simulink model "Two_Zone_MVDC_PSolver_R2020b"  (R2020b)
settings: Solver=FixedStepDiscrete  StartTime=0.0  StopTime=30  FixedStep=TsELEC  RelTol=1e-3  EnableMultiTasking=on
InitFcn:
  | TsELEC = 25e-6;
  | Ts = 25e-6;
  | TsTHERMAL = 1e-3;
  | TsCont = TsELEC;
  | Rsnub = 1e4;
undefined symbols (not defined in the file or in its folder): DiscIntNeverNeededParam, ee_sli_rtmsupport, GABDA, GABDB, GBBDA, GBBDB, gcbh, GPMMA, GPPMB, GPPMC, SADA, SADB, SADC, SADD, SBDA, SBDB, SBDC, SCDA, SCDB, SCDC, SCDD, SDDA, SDDB, SDDC, SDDD, SDDE
libraries: fl_lib x138, nesl_utility x69, ee_lib x52, simulink x3, pid_lib x3, eeTransforms x3, sps_avr x2, powerlib_meascontrol x2, slrealtimetgmanagement x1
(part 1 of 4)
settings Model: SimulationMode=accelerator  Creator=gdudgeon  LastModifiedBy=gdudgeon
settings SolverCC: ConcurrentTasks=on  PositivePriorityOrder=on  AutoInsertRateTranBlk=on
settings DataIOCC: SaveFormat=StructureWithTime  SaveOutput=off  DSMLogging=off  SaveTime=off  ReturnWorkspaceOutputs=off
settings OptimizationCC: BlockReduction=off  OptimizeBlockIOStorage=off  BufferReuse=off  GlobalBufferReuse=off  ExpressionFolding=off  LocalBlockOutputs=off  OptimizeDataStoreBuffers=off  BusAssignmentInplaceUpdate=off
settings HardwareCC: ProdBitPerLong=64  ProdLongLongMode=on  ProdHWDeviceType=Intel->x86-64 (Linux 64)
settings ModelReferenceCC: ModelReferenceNumInstancesAllowed=Single  ModelReferenceMinAlgLoopOccurrences=on
settings SFSimCC: CustomCodeUndefinedFunction=UseInterfaceOnly
settings RTWCC: Description=Simulink Real-Time  SystemTargetFile=slrealtime.tlc  TLCOptions=-axPCMaxOverloads=300  TemplateMakefile=slrealtime_default_tmf  Toolchain=Simulink Real-Time Toolchain  BuildConfiguration=Faster Runs  CodeExecutionProfiling=on  TargetLang=C++

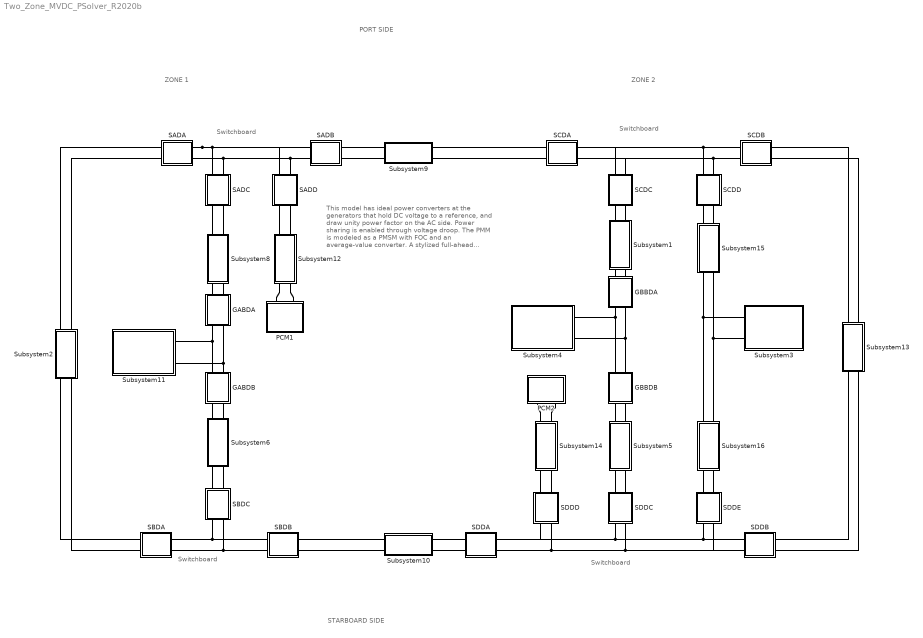
== system Two_Zone_MVDC_PSolver_R2020b ==
  note: This model has ideal power converters at the generators that hold DC voltage to a reference, and draw unity power factor on the AC side. Power sharing is enabled through voltage droop.
      |
      | The PMM is modeled as a PMSM with FOC and an average-value converter.
      |
      | A stylized full-ahead crash-stop maneuver with quadrant II regeneration is simulated.
      |
      | The model uses snubbers on the inductive lines to enable the use of partitioning solver.
  note: PORT SIDE
  note: Switchboard
  note: ZONE 1
  note: ZONE 2
  note: Switchboard
  note: Switchboard
  note: Switchboard
  note: STARBOARD SIDE
  GABDA : Subsystem  mask{status=GABDA}
      mask prompts: status "Initial Status"
      mask init:
      | if ~status
      |     
      |     set(gcbh,'BackgroundColor','green')
      |     
      | elseif status
      |     
      |     set(gcbh,'BackgroundColor','red')
      |     
      | end
  GABDB : Subsystem  mask{status=GABDB}
      mask prompts: status "Initial Status"
      mask init:
      | if ~status
      |     
      |     set(gcbh,'BackgroundColor','green')
      |     
      | elseif status
      |     
      |     set(gcbh,'BackgroundColor','red')
      |     
      | end
  GBBDA : Subsystem  mask{status=GBBDA}
      mask prompts: status "Initial Status"
      mask init:
      | if ~status
      |     
      |     set(gcbh,'BackgroundColor','green')
      |     
      | elseif status
      |     
      |     set(gcbh,'BackgroundColor','red')
      |     
      | end
  GBBDB : Subsystem  mask{status=GBBDB}
      mask prompts: status "Initial Status"
      mask init:
      | if ~status
      |     
      |     set(gcbh,'BackgroundColor','green')
      |     
      | elseif status
      |     
      |     set(gcbh,'BackgroundColor','red')
      |     
      | end
  PCM1 : Subsystem
      mask Display: disp('PCM1')
  PCM2 : Subsystem
      mask Display: disp('PCM2')
  SADA : Subsystem  mask{status=SADA}
      mask prompts: status "Initial Status"
      mask init:
      | if ~status
      |     
      |     set(gcbh,'BackgroundColor','green')
      |     
      | elseif status
      |     
      |     set(gcbh,'BackgroundColor','red')
      |     
      | end
  SADB : Subsystem  mask{status=SADB}
      mask prompts: status "Initial Status"
      mask init:
      | if ~status
      |     
      |     set(gcbh,'BackgroundColor','green')
      |     
      | elseif status
      |     
      |     set(gcbh,'BackgroundColor','red')
      |     
      | end
  SADC : Subsystem  mask{status=SADC}
      mask prompts: status "Initial Status"
      mask init:
      | if ~status
      |     
      |     set(gcbh,'BackgroundColor','green')
      |     
      | elseif status
      |     
      |     set(gcbh,'BackgroundColor','red')
      |     
      | end
  SADD : Subsystem  mask{status=SADD}
      mask prompts: status "Initial Status"
      mask init:
      | if ~status
      |     
      |     set(gcbh,'BackgroundColor','green')
      |     
      | elseif status
      |     
      |     set(gcbh,'BackgroundColor','red')
      |     
      | end
  SBDA : Subsystem  mask{status=SBDA}
      mask prompts: status "Initial Status"
      mask init:
      | if ~status
      |     
      |     set(gcbh,'BackgroundColor','green')
      |     
      | elseif status
      |     
      |     set(gcbh,'BackgroundColor','red')
      |     
      | end
  SBDB : Subsystem  mask{status=SBDB}
      mask prompts: status "Initial Status"
      mask init:
      | if ~status
      |     
      |     set(gcbh,'BackgroundColor','green')
      |     
      | elseif status
      |     
      |     set(gcbh,'BackgroundColor','red')
      |     
      | end
  SBDC : Subsystem  mask{status=SBDC}
      mask prompts: status "Initial Status"
      mask init:
      | if ~status
      |     
      |     set(gcbh,'BackgroundColor','green')
      |     
      | elseif status
      |     
      |     set(gcbh,'BackgroundColor','red')
      |     
      | end
  SCDA : Subsystem  mask{status=SCDA}
      mask prompts: status "Initial Status"
      mask init:
      | if ~status
      |     
      |     set(gcbh,'BackgroundColor','green')
      |     
      | elseif status
      |     
      |     set(gcbh,'BackgroundColor','red')
      |     
      | end
  SCDB : Subsystem  mask{status=SCDB}
      mask prompts: status "Initial Status"
      mask init:
      | if ~status
      |     
      |     set(gcbh,'BackgroundColor','green')
      |     
      | elseif status
      |     
      |     set(gcbh,'BackgroundColor','red')
      |     
      | end
  SCDC : Subsystem  mask{status=SCDC}
      mask prompts: status "Initial Status"
      mask init:
      | if ~status
      |     
      |     set(gcbh,'BackgroundColor','green')
      |     
      | elseif status
      |     
      |     set(gcbh,'BackgroundColor','red')
      |     
      | end
  SCDD : Subsystem  mask{status=SCDD}
      mask prompts: status "Initial Status"
      mask init:
      | if ~status
      |     
      |     set(gcbh,'BackgroundColor','green')
      |     
      | elseif status
      |     
      |     set(gcbh,'BackgroundColor','red')
      |     
      | end
  SDDA : Subsystem  mask{status=SDDA}
      mask prompts: status "Initial Status"
      mask init:
      | if ~status
      |     
      |     set(gcbh,'BackgroundColor','green')
      |     
      | elseif status
      |     
      |     set(gcbh,'BackgroundColor','red')
      |     
      | end
  SDDB : Subsystem  mask{status=SDDB}
      mask prompts: status "Initial Status"
      mask init:
      | if ~status
      |     
      |     set(gcbh,'BackgroundColor','green')
      |     
      | elseif status
      |     
      |     set(gcbh,'BackgroundColor','red')
      |     
      | end
  SDDC : Subsystem  mask{status=SDDC}
      mask prompts: status "Initial Status"
      mask init:
      | if ~status
      |     
      |     set(gcbh,'BackgroundColor','green')
      |     
      | elseif status
      |     
      |     set(gcbh,'BackgroundColor','red')
      |     
      | end
  SDDD : Subsystem  mask{status=SDDD}
      mask prompts: status "Initial Status"
      mask init:
      | if ~status
      |     
      |     set(gcbh,'BackgroundColor','green')
      |     
      | elseif status
      |     
      |     set(gcbh,'BackgroundColor','red')
      |     
      | end
  SDDE : Subsystem  mask{status=SDDE}
      mask prompts: status "Initial Status"
      mask init:
      | if ~status
      |     
      |     set(gcbh,'BackgroundColor','green')
      |     
      | elseif status
      |     
      |     set(gcbh,'BackgroundColor','red')
      |     
      | end
  Subsystem1 : Subsystem
      mask Display: disp('CS11*')
  Subsystem10 : Subsystem
      mask Display: disp('CS6')
  Subsystem11 : Subsystem
      mask Display: disp('PGM1')
  Subsystem12 : Subsystem
      mask Display: disp('CS21')
  Subsystem13 : Subsystem
      mask Display: disp('CS4')
  Subsystem14 : Subsystem
      mask Display: disp('CS22')
  Subsystem15 : Subsystem
      mask Display: disp('CS14*')
  Subsystem16 : Subsystem
      mask Display: disp('CS14')
  Subsystem2 : Subsystem
      mask Display: disp('CS8')
  Subsystem3 : Subsystem
      mask Display: disp('PMM')
  Subsystem4 : Subsystem
      mask Display: disp('PGM2')
  Subsystem5 : Subsystem
      mask Display: disp('CS11')
  Subsystem6 : Subsystem
      mask Display: disp('CS9*')
  Subsystem8 : Subsystem
      mask Display: disp('CS9')
  Subsystem9 : Subsystem
      mask Display: disp('CS2')
  connections:
  SADA/RConn2 -- SADC/LConn2 -- SADD/LConn2 -- SADB/LConn2
  SBDC/RConn2 -- SBDB/LConn2 -- SBDA/RConn2
  Subsystem11/RConn2 -- GABDB/LConn2 -- GABDA/RConn2
  Subsystem11/RConn1 -- GABDB/LConn1 -- GABDA/RConn1
  SADA/RConn1 -- SADD/LConn1 -- SADB/LConn1 -- SADC/LConn1
  SBDC/RConn1 -- SBDB/LConn1 -- SBDA/RConn1
  SCDA/LConn2 -- Subsystem9/LConn2
  SADB/RConn1 -- Subsystem9/RConn1
  Subsystem12/LConn1 -- SADD/RConn1
  SBDA/LConn2 -- Subsystem2/RConn2
  SBDC/LConn1 -- Subsystem6/RConn1
  Subsystem12/RConn1 -- PCM1/LConn1
  SBDB/RConn1 -- Subsystem10/RConn1
  SBDC/LConn2 -- Subsystem6/RConn2
  Subsystem2/LConn1 -- SADA/LConn1
  Subsystem12/RConn2 -- PCM1/LConn2
  Subsystem12/LConn2 -- SADD/RConn2
  SADC/RConn1 -- Subsystem8/LConn1
  SBDB/RConn2 -- Subsystem10/RConn2
  SADB/RConn2 -- Subsystem9/RConn2
  Subsystem2/LConn2 -- SADA/LConn2
  SBDA/LConn1 -- Subsystem2/RConn1
  SADC/RConn2 -- Subsystem8/LConn2
  GBBDA/RConn1 -- GBBDB/LConn1 -- Subsystem4/RConn1
  SDDC/RConn2 -- SDDB/LConn2 -- SDDE/RConn2 -- SDDA/RConn2 -- SDDD/RConn2
  SCDC/LConn2 -- SCDA/RConn2 -- SCDD/LConn2 -- SCDB/LConn2
  SDDC/RConn1 -- SDDA/RConn1 -- SDDD/RConn1 -- SDDB/LConn1 -- SDDE/RConn1
  SCDC/LConn1 -- SCDA/RConn1 -- SCDD/LConn1 -- SCDB/LConn1
  GBBDA/RConn2 -- GBBDB/LConn2 -- Subsystem4/RConn2
  SCDC/RConn2 -- Subsystem1/LConn2
  SCDB/RConn1 -- Subsystem13/LConn1
  SDDB/RConn1 -- Subsystem13/RConn1
  SDDC/LConn2 -- Subsystem5/RConn2
  SDDB/RConn2 -- Subsystem13/RConn2
  SCDB/RConn2 -- Subsystem13/LConn2
  SDDC/LConn1 -- Subsystem5/RConn1
  SCDC/RConn1 -- Subsystem1/LConn1
  Subsystem9/LConn1 -- SCDA/LConn1
  Subsystem10/LConn1 -- SDDA/LConn1
  Subsystem10/LConn2 -- SDDA/LConn2
  GBBDA/LConn1 -- Subsystem1/RConn1
  GBBDA/LConn2 -- Subsystem1/RConn2
  GBBDB/RConn1 -- Subsystem5/LConn1
  GBBDB/RConn2 -- Subsystem5/LConn2
  GABDA/LConn1 -- Subsystem8/RConn1
  GABDA/LConn2 -- Subsystem8/RConn2
  GABDB/RConn1 -- Subsystem6/LConn1
  GABDB/RConn2 -- Subsystem6/LConn2
  Subsystem14/LConn1 -- PCM2/LConn1
  Subsystem14/LConn2 -- PCM2/LConn2
  Subsystem14/RConn1 -- SDDD/LConn1
  Subsystem14/RConn2 -- SDDD/LConn2
  Subsystem15/LConn2 -- SCDD/RConn2
  Subsystem15/LConn1 -- SCDD/RConn1
  Subsystem16/RConn1 -- SDDE/LConn1
  Subsystem16/RConn2 -- SDDE/LConn2
  Subsystem16/LConn1 -- Subsystem3/LConn1 -- Subsystem15/RConn1
  Subsystem15/RConn2 -- Subsystem16/LConn2 -- Subsystem3/LConn2

== system Two_Zone_MVDC_PSolver_R2020b/GABDA ==
  GABDA : ee_lib/Switches & Breakers/DPST Switch  R_closed=1e-4 Ohm  G_open=1e-6 S  Threshold=0.5 V  Width=0 V  model_dynamics=0  t_on=1e-3 s  t_off=1e-3 s  initial_vT=0 V
      settings: SourceProductBaseCode=PS  InternalSimscapePortConfiguration="{\"Bottom\":[],\"Left\":[{\"id\":\"vT\",\"label\":\"vT\",\"type\":\"input\"},{\"id\":\"p1\",\"label\":\"\",\"type\":\"foundation.electrical.electrical\"},{\"id\":\"p2\",\"label\":\"\",\"type\":\"foundation.electrical.electrical\"}],\"Right\":[{\"id\":\"n1\",\"label\":\"\",\"type\":\"foundation.electrical.electrical\"},{\"id\":\"n2\",\"label\":\"\",\"type\":\"foundation.electrical.electrical\"}],\"Top\":[]}"
  Simulink-PS Converter : nesl_utility/Simulink-PS Converter  PhysicalDomain=network_engine_domain  SubClassName=ps_input  LeftPortType=input  RightPortType=output  PseudoPeriodic=off  Frequencies=[]  NoiseDistribution=none  NoiseParameters=[]  Unit=1  AffineConversion=off  FilteringAndDerivatives=provide  SimscapeFilterOrder=1  InputFilterTimeConstant=0.001  UdotUserProvided=0
  "+ " : PMIOPort  Side=Right
  + : PMIOPort  Port=2  Side=Left
  "- " : PMIOPort  Port=3  Side=Right
  - : PMIOPort  Port=4  Side=Left
  wires:
  [GABDA] -> Simulink-PS Converter/1
  connections:
  GABDA/RConn1 -- "+ "/RConn1
  GABDA/LConn3 -- -/RConn1
  GABDA/RConn2 -- "- "/RConn1
  Simulink-PS Converter/RConn1 -- GABDA/LConn1
  GABDA/LConn2 -- +/RConn1

== system Two_Zone_MVDC_PSolver_R2020b/GABDB ==
  GABDB : ee_lib/Switches & Breakers/DPST Switch  R_closed=1e-4 Ohm  G_open=1e-6 S  Threshold=0.5 V  Width=0 V  model_dynamics=0  t_on=1e-3 s  t_off=1e-3 s  initial_vT=0 V
      settings: SourceProductBaseCode=PS  InternalSimscapePortConfiguration="{\"Bottom\":[],\"Left\":[{\"id\":\"vT\",\"label\":\"vT\",\"type\":\"input\"},{\"id\":\"p1\",\"label\":\"\",\"type\":\"foundation.electrical.electrical\"},{\"id\":\"p2\",\"label\":\"\",\"type\":\"foundation.electrical.electrical\"}],\"Right\":[{\"id\":\"n1\",\"label\":\"\",\"type\":\"foundation.electrical.electrical\"},{\"id\":\"n2\",\"label\":\"\",\"type\":\"foundation.electrical.electrical\"}],\"Top\":[]}"
  Simulink-PS Converter : nesl_utility/Simulink-PS Converter  PhysicalDomain=network_engine_domain  SubClassName=ps_input  LeftPortType=input  RightPortType=output  PseudoPeriodic=off  Frequencies=[]  NoiseDistribution=none  NoiseParameters=[]  Unit=1  AffineConversion=off  FilteringAndDerivatives=provide  SimscapeFilterOrder=1  InputFilterTimeConstant=0.001  UdotUserProvided=0
  "+ " : PMIOPort  Side=Right
  + : PMIOPort  Port=2  Side=Left
  "- " : PMIOPort  Port=3  Side=Right
  - : PMIOPort  Port=4  Side=Left
  wires:
  [GABDB] -> Simulink-PS Converter/1
  connections:
  GABDB/LConn2 -- +/RConn1
  Simulink-PS Converter/RConn1 -- GABDB/LConn1
  GABDB/RConn2 -- "- "/RConn1
  GABDB/LConn3 -- -/RConn1
  GABDB/RConn1 -- "+ "/RConn1

== system Two_Zone_MVDC_PSolver_R2020b/GBBDA ==
  GBBDA : ee_lib/Switches & Breakers/DPST Switch  R_closed=1e-4 Ohm  G_open=1e-6 S  Threshold=0.5 V  Width=0 V  model_dynamics=0  t_on=1e-3 s  t_off=1e-3 s  initial_vT=0 V
      settings: SourceProductBaseCode=PS  InternalSimscapePortConfiguration="{\"Bottom\":[],\"Left\":[{\"id\":\"vT\",\"label\":\"vT\",\"type\":\"input\"},{\"id\":\"p1\",\"label\":\"\",\"type\":\"foundation.electrical.electrical\"},{\"id\":\"p2\",\"label\":\"\",\"type\":\"foundation.electrical.electrical\"}],\"Right\":[{\"id\":\"n1\",\"label\":\"\",\"type\":\"foundation.electrical.electrical\"},{\"id\":\"n2\",\"label\":\"\",\"type\":\"foundation.electrical.electrical\"}],\"Top\":[]}"
  Simulink-PS Converter : nesl_utility/Simulink-PS Converter  PhysicalDomain=network_engine_domain  SubClassName=ps_input  LeftPortType=input  RightPortType=output  PseudoPeriodic=off  Frequencies=[]  NoiseDistribution=none  NoiseParameters=[]  Unit=1  AffineConversion=off  FilteringAndDerivatives=provide  SimscapeFilterOrder=1  InputFilterTimeConstant=0.001  UdotUserProvided=0
  "+ " : PMIOPort  Side=Right
  + : PMIOPort  Port=2  Side=Left
  "- " : PMIOPort  Port=3  Side=Right
  - : PMIOPort  Port=4  Side=Left
  wires:
  [GBBDA] -> Simulink-PS Converter/1
  connections:
  GBBDA/RConn1 -- "+ "/RConn1
  GBBDA/LConn3 -- -/RConn1
  GBBDA/RConn2 -- "- "/RConn1
  Simulink-PS Converter/RConn1 -- GBBDA/LConn1
  GBBDA/LConn2 -- +/RConn1

== system Two_Zone_MVDC_PSolver_R2020b/GBBDB ==
  GBBDB : ee_lib/Switches & Breakers/DPST Switch  R_closed=1e-4 Ohm  G_open=1e-6 S  Threshold=0.5 V  Width=0 V  model_dynamics=0  t_on=1e-3 s  t_off=1e-3 s  initial_vT=0 V
      settings: SourceProductBaseCode=PS  InternalSimscapePortConfiguration="{\"Bottom\":[],\"Left\":[{\"id\":\"vT\",\"label\":\"vT\",\"type\":\"input\"},{\"id\":\"p1\",\"label\":\"\",\"type\":\"foundation.electrical.electrical\"},{\"id\":\"p2\",\"label\":\"\",\"type\":\"foundation.electrical.electrical\"}],\"Right\":[{\"id\":\"n1\",\"label\":\"\",\"type\":\"foundation.electrical.electrical\"},{\"id\":\"n2\",\"label\":\"\",\"type\":\"foundation.electrical.electrical\"}],\"Top\":[]}"
  Simulink-PS Converter : nesl_utility/Simulink-PS Converter  PhysicalDomain=network_engine_domain  SubClassName=ps_input  LeftPortType=input  RightPortType=output  PseudoPeriodic=off  Frequencies=[]  NoiseDistribution=none  NoiseParameters=[]  Unit=1  AffineConversion=off  FilteringAndDerivatives=provide  SimscapeFilterOrder=1  InputFilterTimeConstant=0.001  UdotUserProvided=0
  "+ " : PMIOPort  Side=Right
  + : PMIOPort  Port=2  Side=Left
  "- " : PMIOPort  Port=3  Side=Right
  - : PMIOPort  Port=4  Side=Left
  wires:
  [GBBDB] -> Simulink-PS Converter/1
  connections:
  GBBDB/LConn2 -- +/RConn1
  Simulink-PS Converter/RConn1 -- GBBDB/LConn1
  GBBDB/RConn2 -- "- "/RConn1
  GBBDB/LConn3 -- -/RConn1
  GBBDB/RConn1 -- "+ "/RConn1

== system Two_Zone_MVDC_PSolver_R2020b/PCM1 ==
  Bus Creator : BusCreator  Inputs=3
  Current Sensor : fl_lib/Electrical/Electrical Sensors/Current Sensor
  PS-Simulink Converter : nesl_utility/PS-Simulink Converter  PhysicalDomain=network_engine_domain  SubClassName=ps_output  LeftPortType=input  RightPortType=output  PseudoPeriodic=off  Frequencies=[]  Unit=1  AffineConversion=off
  PS-Simulink Converter1 : nesl_utility/PS-Simulink Converter  PhysicalDomain=network_engine_domain  SubClassName=ps_output  LeftPortType=input  RightPortType=output  PseudoPeriodic=off  Frequencies=[]  Unit=1  AffineConversion=off
  Product : Product
  Resistor : fl_lib/Electrical/Electrical Elements/Resistor  R=100 Ohm  i_specify=off  i_priority=None  i=0 A  i_nominal_specify=off  i_nominal_unit=A  i_nominal_value=1  v_specify=off  v_priority=None  v=0 V  v_nominal_specify=off  v_nominal_unit=V  v_nominal_value=1
  Terminator : Terminator
  Voltage Sensor : fl_lib/Electrical/Electrical Sensors/Voltage Sensor
  + : PMIOPort  Side=Left
  - : PMIOPort  Port=2  Side=Left
  wires:
  Bus Creator/1 -> Terminator/1  "PCM1"
  Product/1 -> Bus Creator/3  "P"
  PS-Simulink Converter1/1 -> Bus Creator/2, Product/2  "V"
  PS-Simulink Converter/1 -> Bus Creator/1, Product/1  "I"
  connections:
  Current Sensor/LConn1 -- +/RConn1
  Voltage Sensor/RConn1 -- PS-Simulink Converter1/LConn1
  PS-Simulink Converter/LConn1 -- Current Sensor/RConn1
  Resistor/RConn1 -- -/RConn1 -- Voltage Sensor/RConn2
  Voltage Sensor/LConn1 -- Resistor/LConn1 -- Current Sensor/RConn2

== system Two_Zone_MVDC_PSolver_R2020b/PCM2 ==
  Bus Creator : BusCreator  Inputs=3
  Current Sensor : fl_lib/Electrical/Electrical Sensors/Current Sensor
  PS-Simulink Converter : nesl_utility/PS-Simulink Converter  PhysicalDomain=network_engine_domain  SubClassName=ps_output  LeftPortType=input  RightPortType=output  PseudoPeriodic=off  Frequencies=[]  Unit=1  AffineConversion=off
  PS-Simulink Converter1 : nesl_utility/PS-Simulink Converter  PhysicalDomain=network_engine_domain  SubClassName=ps_output  LeftPortType=input  RightPortType=output  PseudoPeriodic=off  Frequencies=[]  Unit=1  AffineConversion=off
  Product : Product
  Resistor : fl_lib/Electrical/Electrical Elements/Resistor  R=100 Ohm  i_specify=off  i_priority=None  i=0 A  i_nominal_specify=off  i_nominal_unit=A  i_nominal_value=1  v_specify=off  v_priority=None  v=0 V  v_nominal_specify=off  v_nominal_unit=V  v_nominal_value=1
  Terminator : Terminator
  Voltage Sensor : fl_lib/Electrical/Electrical Sensors/Voltage Sensor
  + : PMIOPort  Side=Left
  - : PMIOPort  Port=2  Side=Left
  wires:
  Bus Creator/1 -> Terminator/1  "PCM2"
  Product/1 -> Bus Creator/3  "P"
  PS-Simulink Converter1/1 -> Bus Creator/2, Product/2  "V"
  PS-Simulink Converter/1 -> Bus Creator/1, Product/1  "I"
  connections:
  +/RConn1 -- Current Sensor/LConn1
  Voltage Sensor/RConn1 -- PS-Simulink Converter1/LConn1
  PS-Simulink Converter/LConn1 -- Current Sensor/RConn1
  Resistor/RConn1 -- -/RConn1 -- Voltage Sensor/RConn2
  Voltage Sensor/LConn1 -- Resistor/LConn1 -- Current Sensor/RConn2

== system Two_Zone_MVDC_PSolver_R2020b/SADA ==
  SADA : ee_lib/Switches & Breakers/DPST Switch  R_closed=1e-4 Ohm  G_open=1e-6 S  Threshold=0.5 V  Width=0 V  model_dynamics=0  t_on=1e-3 s  t_off=1e-3 s  initial_vT=0 V
      settings: SourceProductBaseCode=PS  InternalSimscapePortConfiguration="{\"Bottom\":[],\"Left\":[{\"id\":\"vT\",\"label\":\"vT\",\"type\":\"input\"},{\"id\":\"p1\",\"label\":\"\",\"type\":\"foundation.electrical.electrical\"},{\"id\":\"p2\",\"label\":\"\",\"type\":\"foundation.electrical.electrical\"}],\"Right\":[{\"id\":\"n1\",\"label\":\"\",\"type\":\"foundation.electrical.electrical\"},{\"id\":\"n2\",\"label\":\"\",\"type\":\"foundation.electrical.electrical\"}],\"Top\":[]}"
  Simulink-PS Converter : nesl_utility/Simulink-PS Converter  PhysicalDomain=network_engine_domain  SubClassName=ps_input  LeftPortType=input  RightPortType=output  PseudoPeriodic=off  Frequencies=[]  NoiseDistribution=none  NoiseParameters=[]  Unit=1  AffineConversion=off  FilteringAndDerivatives=provide  SimscapeFilterOrder=1  InputFilterTimeConstant=0.001  UdotUserProvided=0
  "+ " : PMIOPort  Side=Right
  + : PMIOPort  Port=2  Side=Left
  "- " : PMIOPort  Port=3  Side=Right
  - : PMIOPort  Port=4  Side=Left
  wires:
  [SADA] -> Simulink-PS Converter/1
  connections:
  SADA/RConn1 -- "+ "/RConn1
  SADA/LConn3 -- -/RConn1
  SADA/RConn2 -- "- "/RConn1
  Simulink-PS Converter/RConn1 -- SADA/LConn1
  SADA/LConn2 -- +/RConn1

== system Two_Zone_MVDC_PSolver_R2020b/SADB ==
  SADB : ee_lib/Switches & Breakers/DPST Switch  R_closed=1e-4 Ohm  G_open=1e-6 S  Threshold=0.5 V  Width=0 V  model_dynamics=0  t_on=1e-3 s  t_off=1e-3 s  initial_vT=0 V
      settings: SourceProductBaseCode=PS  InternalSimscapePortConfiguration="{\"Bottom\":[],\"Left\":[{\"id\":\"vT\",\"label\":\"vT\",\"type\":\"input\"},{\"id\":\"p1\",\"label\":\"\",\"type\":\"foundation.electrical.electrical\"},{\"id\":\"p2\",\"label\":\"\",\"type\":\"foundation.electrical.electrical\"}],\"Right\":[{\"id\":\"n1\",\"label\":\"\",\"type\":\"foundation.electrical.electrical\"},{\"id\":\"n2\",\"label\":\"\",\"type\":\"foundation.electrical.electrical\"}],\"Top\":[]}"
  Simulink-PS Converter : nesl_utility/Simulink-PS Converter  PhysicalDomain=network_engine_domain  SubClassName=ps_input  LeftPortType=input  RightPortType=output  PseudoPeriodic=off  Frequencies=[]  NoiseDistribution=none  NoiseParameters=[]  Unit=1  AffineConversion=off  FilteringAndDerivatives=provide  SimscapeFilterOrder=1  InputFilterTimeConstant=0.001  UdotUserProvided=0
  "+ " : PMIOPort  Side=Right
  + : PMIOPort  Port=2  Side=Left
  "- " : PMIOPort  Port=3  Side=Right
  - : PMIOPort  Port=4  Side=Left
  wires:
  [SADB] -> Simulink-PS Converter/1
  connections:
  SADB/LConn2 -- +/RConn1
  Simulink-PS Converter/RConn1 -- SADB/LConn1
  SADB/RConn2 -- "- "/RConn1
  SADB/LConn3 -- -/RConn1
  SADB/RConn1 -- "+ "/RConn1

== system Two_Zone_MVDC_PSolver_R2020b/SADC ==
  SADC : ee_lib/Switches & Breakers/DPST Switch  R_closed=1e-4 Ohm  G_open=1e-6 S  Threshold=0.5 V  Width=0 V  model_dynamics=0  t_on=1e-3 s  t_off=1e-3 s  initial_vT=0 V
      settings: SourceProductBaseCode=PS  InternalSimscapePortConfiguration="{\"Bottom\":[],\"Left\":[{\"id\":\"vT\",\"label\":\"vT\",\"type\":\"input\"},{\"id\":\"p1\",\"label\":\"\",\"type\":\"foundation.electrical.electrical\"},{\"id\":\"p2\",\"label\":\"\",\"type\":\"foundation.electrical.electrical\"}],\"Right\":[{\"id\":\"n1\",\"label\":\"\",\"type\":\"foundation.electrical.electrical\"},{\"id\":\"n2\",\"label\":\"\",\"type\":\"foundation.electrical.electrical\"}],\"Top\":[]}"
  Simulink-PS Converter : nesl_utility/Simulink-PS Converter  PhysicalDomain=network_engine_domain  SubClassName=ps_input  LeftPortType=input  RightPortType=output  PseudoPeriodic=off  Frequencies=[]  NoiseDistribution=none  NoiseParameters=[]  Unit=1  AffineConversion=off  FilteringAndDerivatives=provide  SimscapeFilterOrder=1  InputFilterTimeConstant=0.001  UdotUserProvided=0
  "+ " : PMIOPort  Side=Right
  + : PMIOPort  Port=2  Side=Left
  "- " : PMIOPort  Port=3  Side=Right
  - : PMIOPort  Port=4  Side=Left
  wires:
  [SADC] -> Simulink-PS Converter/1
  connections:
  SADC/LConn2 -- +/RConn1
  Simulink-PS Converter/RConn1 -- SADC/LConn1
  SADC/RConn2 -- "- "/RConn1
  SADC/LConn3 -- -/RConn1
  SADC/RConn1 -- "+ "/RConn1

== system Two_Zone_MVDC_PSolver_R2020b/SADD ==
  SADD : ee_lib/Switches & Breakers/DPST Switch  R_closed=1e-4 Ohm  G_open=1e-6 S  Threshold=0.5 V  Width=0 V  model_dynamics=0  t_on=1e-3 s  t_off=1e-3 s  initial_vT=0 V
      settings: SourceProductBaseCode=PS  InternalSimscapePortConfiguration="{\"Bottom\":[],\"Left\":[{\"id\":\"vT\",\"label\":\"vT\",\"type\":\"input\"},{\"id\":\"p1\",\"label\":\"\",\"type\":\"foundation.electrical.electrical\"},{\"id\":\"p2\",\"label\":\"\",\"type\":\"foundation.electrical.electrical\"}],\"Right\":[{\"id\":\"n1\",\"label\":\"\",\"type\":\"foundation.electrical.electrical\"},{\"id\":\"n2\",\"label\":\"\",\"type\":\"foundation.electrical.electrical\"}],\"Top\":[]}"
  Simulink-PS Converter : nesl_utility/Simulink-PS Converter  PhysicalDomain=network_engine_domain  SubClassName=ps_input  LeftPortType=input  RightPortType=output  PseudoPeriodic=off  Frequencies=[]  NoiseDistribution=none  NoiseParameters=[]  Unit=1  AffineConversion=off  FilteringAndDerivatives=provide  SimscapeFilterOrder=1  InputFilterTimeConstant=0.001  UdotUserProvided=0
  "+ " : PMIOPort  Side=Right
  + : PMIOPort  Port=2  Side=Left
  "- " : PMIOPort  Port=3  Side=Right
  - : PMIOPort  Port=4  Side=Left
  wires:
  [SADD] -> Simulink-PS Converter/1
  connections:
  SADD/RConn1 -- "+ "/RConn1
  SADD/LConn3 -- -/RConn1
  SADD/RConn2 -- "- "/RConn1
  Simulink-PS Converter/RConn1 -- SADD/LConn1
  SADD/LConn2 -- +/RConn1

== system Two_Zone_MVDC_PSolver_R2020b/SBDA ==
  SBDA : ee_lib/Switches & Breakers/DPST Switch  R_closed=1e-4 Ohm  G_open=1e-6 S  Threshold=0.5 V  Width=0 V  model_dynamics=0  t_on=1e-3 s  t_off=1e-3 s  initial_vT=0 V
      settings: SourceProductBaseCode=PS  InternalSimscapePortConfiguration="{\"Bottom\":[],\"Left\":[{\"id\":\"vT\",\"label\":\"vT\",\"type\":\"input\"},{\"id\":\"p1\",\"label\":\"\",\"type\":\"foundation.electrical.electrical\"},{\"id\":\"p2\",\"label\":\"\",\"type\":\"foundation.electrical.electrical\"}],\"Right\":[{\"id\":\"n1\",\"label\":\"\",\"type\":\"foundation.electrical.electrical\"},{\"id\":\"n2\",\"label\":\"\",\"type\":\"foundation.electrical.electrical\"}],\"Top\":[]}"
  Simulink-PS Converter : nesl_utility/Simulink-PS Converter  PhysicalDomain=network_engine_domain  SubClassName=ps_input  LeftPortType=input  RightPortType=output  PseudoPeriodic=off  Frequencies=[]  NoiseDistribution=none  NoiseParameters=[]  Unit=1  AffineConversion=off  FilteringAndDerivatives=provide  SimscapeFilterOrder=1  InputFilterTimeConstant=0.001  UdotUserProvided=0
  "+ " : PMIOPort  Side=Right
  + : PMIOPort  Port=2  Side=Left
  "- " : PMIOPort  Port=3  Side=Right
  - : PMIOPort  Port=4  Side=Left
  wires:
  [SBDA] -> Simulink-PS Converter/1
  connections:
  SBDA/LConn2 -- +/RConn1
  Simulink-PS Converter/RConn1 -- SBDA/LConn1
  SBDA/RConn2 -- "- "/RConn1
  SBDA/LConn3 -- -/RConn1
  SBDA/RConn1 -- "+ "/RConn1

== system Two_Zone_MVDC_PSolver_R2020b/SBDB ==
  SBDB : ee_lib/Switches & Breakers/DPST Switch  R_closed=1e-4 Ohm  G_open=1e-6 S  Threshold=0.5 V  Width=0 V  model_dynamics=0  t_on=1e-3 s  t_off=1e-3 s  initial_vT=0 V
      settings: SourceProductBaseCode=PS  InternalSimscapePortConfiguration="{\"Bottom\":[],\"Left\":[{\"id\":\"vT\",\"label\":\"vT\",\"type\":\"input\"},{\"id\":\"p1\",\"label\":\"\",\"type\":\"foundation.electrical.electrical\"},{\"id\":\"p2\",\"label\":\"\",\"type\":\"foundation.electrical.electrical\"}],\"Right\":[{\"id\":\"n1\",\"label\":\"\",\"type\":\"foundation.electrical.electrical\"},{\"id\":\"n2\",\"label\":\"\",\"type\":\"foundation.electrical.electrical\"}],\"Top\":[]}"
  Simulink-PS Converter : nesl_utility/Simulink-PS Converter  PhysicalDomain=network_engine_domain  SubClassName=ps_input  LeftPortType=input  RightPortType=output  PseudoPeriodic=off  Frequencies=[]  NoiseDistribution=none  NoiseParameters=[]  Unit=1  AffineConversion=off  FilteringAndDerivatives=provide  SimscapeFilterOrder=1  InputFilterTimeConstant=0.001  UdotUserProvided=0
  "+ " : PMIOPort  Side=Right
  + : PMIOPort  Port=2  Side=Left
  "- " : PMIOPort  Port=3  Side=Right
  - : PMIOPort  Port=4  Side=Left
  wires:
  [SBDB] -> Simulink-PS Converter/1
  connections:
  SBDB/RConn1 -- "+ "/RConn1
  SBDB/LConn3 -- -/RConn1
  SBDB/RConn2 -- "- "/RConn1
  Simulink-PS Converter/RConn1 -- SBDB/LConn1
  SBDB/LConn2 -- +/RConn1

== system Two_Zone_MVDC_PSolver_R2020b/SBDC ==
  SBDC : ee_lib/Switches & Breakers/DPST Switch  R_closed=1e-4 Ohm  G_open=1e-6 S  Threshold=0.5 V  Width=0 V  model_dynamics=0  t_on=1e-3 s  t_off=1e-3 s  initial_vT=0 V
      settings: SourceProductBaseCode=PS  InternalSimscapePortConfiguration="{\"Bottom\":[],\"Left\":[{\"id\":\"vT\",\"label\":\"vT\",\"type\":\"input\"},{\"id\":\"p1\",\"label\":\"\",\"type\":\"foundation.electrical.electrical\"},{\"id\":\"p2\",\"label\":\"\",\"type\":\"foundation.electrical.electrical\"}],\"Right\":[{\"id\":\"n1\",\"label\":\"\",\"type\":\"foundation.electrical.electrical\"},{\"id\":\"n2\",\"label\":\"\",\"type\":\"foundation.electrical.electrical\"}],\"Top\":[]}"
  Simulink-PS Converter : nesl_utility/Simulink-PS Converter  PhysicalDomain=network_engine_domain  SubClassName=ps_input  LeftPortType=input  RightPortType=output  PseudoPeriodic=off  Frequencies=[]  NoiseDistribution=none  NoiseParameters=[]  Unit=1  AffineConversion=off  FilteringAndDerivatives=provide  SimscapeFilterOrder=1  InputFilterTimeConstant=0.001  UdotUserProvided=0
  "+ " : PMIOPort  Side=Right
  + : PMIOPort  Port=2  Side=Left
  "- " : PMIOPort  Port=3  Side=Right
  - : PMIOPort  Port=4  Side=Left
  wires:
  [SBDC] -> Simulink-PS Converter/1
  connections:
  SBDC/LConn2 -- +/RConn1
  Simulink-PS Converter/RConn1 -- SBDC/LConn1
  SBDC/RConn2 -- "- "/RConn1
  SBDC/LConn3 -- -/RConn1
  SBDC/RConn1 -- "+ "/RConn1

== system Two_Zone_MVDC_PSolver_R2020b/SCDA ==
  SADA : ee_lib/Switches & Breakers/DPST Switch  R_closed=1e-4 Ohm  G_open=1e-6 S  Threshold=0.5 V  Width=0 V  model_dynamics=0  t_on=1e-3 s  t_off=1e-3 s  initial_vT=0 V
      settings: SourceProductBaseCode=PS  InternalSimscapePortConfiguration="{\"Bottom\":[],\"Left\":[{\"id\":\"vT\",\"label\":\"vT\",\"type\":\"input\"},{\"id\":\"p1\",\"label\":\"\",\"type\":\"foundation.electrical.electrical\"},{\"id\":\"p2\",\"label\":\"\",\"type\":\"foundation.electrical.electrical\"}],\"Right\":[{\"id\":\"n1\",\"label\":\"\",\"type\":\"foundation.electrical.electrical\"},{\"id\":\"n2\",\"label\":\"\",\"type\":\"foundation.electrical.electrical\"}],\"Top\":[]}"
  Simulink-PS Converter : nesl_utility/Simulink-PS Converter  PhysicalDomain=network_engine_domain  SubClassName=ps_input  LeftPortType=input  RightPortType=output  PseudoPeriodic=off  Frequencies=[]  NoiseDistribution=none  NoiseParameters=[]  Unit=1  AffineConversion=off  FilteringAndDerivatives=provide  SimscapeFilterOrder=1  InputFilterTimeConstant=0.001  UdotUserProvided=0
  "+ " : PMIOPort  Side=Right
  + : PMIOPort  Port=2  Side=Left
  "- " : PMIOPort  Port=3  Side=Right
  - : PMIOPort  Port=4  Side=Left
  wires:
  [SCDA] -> Simulink-PS Converter/1
  connections:
  SADA/RConn1 -- "+ "/RConn1
  SADA/LConn3 -- -/RConn1
  SADA/RConn2 -- "- "/RConn1
  Simulink-PS Converter/RConn1 -- SADA/LConn1
  SADA/LConn2 -- +/RConn1

== system Two_Zone_MVDC_PSolver_R2020b/SCDB ==
  SCDB : ee_lib/Switches & Breakers/DPST Switch  R_closed=1e-4 Ohm  G_open=1e-6 S  Threshold=0.5 V  Width=0 V  model_dynamics=0  t_on=1e-3 s  t_off=1e-3 s  initial_vT=0 V
      settings: SourceProductBaseCode=PS  InternalSimscapePortConfiguration="{\"Bottom\":[],\"Left\":[{\"id\":\"vT\",\"label\":\"vT\",\"type\":\"input\"},{\"id\":\"p1\",\"label\":\"\",\"type\":\"foundation.electrical.electrical\"},{\"id\":\"p2\",\"label\":\"\",\"type\":\"foundation.electrical.electrical\"}],\"Right\":[{\"id\":\"n1\",\"label\":\"\",\"type\":\"foundation.electrical.electrical\"},{\"id\":\"n2\",\"label\":\"\",\"type\":\"foundation.electrical.electrical\"}],\"Top\":[]}"
  Simulink-PS Converter : nesl_utility/Simulink-PS Converter  PhysicalDomain=network_engine_domain  SubClassName=ps_input  LeftPortType=input  RightPortType=output  PseudoPeriodic=off  Frequencies=[]  NoiseDistribution=none  NoiseParameters=[]  Unit=1  AffineConversion=off  FilteringAndDerivatives=provide  SimscapeFilterOrder=1  InputFilterTimeConstant=0.001  UdotUserProvided=0
  "+ " : PMIOPort  Side=Right
  + : PMIOPort  Port=2  Side=Left
  "- " : PMIOPort  Port=3  Side=Right
  - : PMIOPort  Port=4  Side=Left
  wires:
  [SCDB] -> Simulink-PS Converter/1
  connections:
  SCDB/LConn2 -- +/RConn1
  Simulink-PS Converter/RConn1 -- SCDB/LConn1
  SCDB/RConn2 -- "- "/RConn1
  SCDB/LConn3 -- -/RConn1
  SCDB/RConn1 -- "+ "/RConn1

== system Two_Zone_MVDC_PSolver_R2020b/SCDC ==
  SADA : ee_lib/Switches & Breakers/DPST Switch  R_closed=1e-4 Ohm  G_open=1e-6 S  Threshold=0.5 V  Width=0 V  model_dynamics=0  t_on=1e-3 s  t_off=1e-3 s  initial_vT=0 V
      settings: SourceProductBaseCode=PS  InternalSimscapePortConfiguration="{\"Bottom\":[],\"Left\":[{\"id\":\"vT\",\"label\":\"vT\",\"type\":\"input\"},{\"id\":\"p1\",\"label\":\"\",\"type\":\"foundation.electrical.electrical\"},{\"id\":\"p2\",\"label\":\"\",\"type\":\"foundation.electrical.electrical\"}],\"Right\":[{\"id\":\"n1\",\"label\":\"\",\"type\":\"foundation.electrical.electrical\"},{\"id\":\"n2\",\"label\":\"\",\"type\":\"foundation.electrical.electrical\"}],\"Top\":[]}"
  Simulink-PS Converter : nesl_utility/Simulink-PS Converter  PhysicalDomain=network_engine_domain  SubClassName=ps_input  LeftPortType=input  RightPortType=output  PseudoPeriodic=off  Frequencies=[]  NoiseDistribution=none  NoiseParameters=[]  Unit=1  AffineConversion=off  FilteringAndDerivatives=provide  SimscapeFilterOrder=1  InputFilterTimeConstant=0.001  UdotUserProvided=0
  "+ " : PMIOPort  Side=Right
  + : PMIOPort  Port=2  Side=Left
  "- " : PMIOPort  Port=3  Side=Right
  - : PMIOPort  Port=4  Side=Left
  wires:
  [SCDC] -> Simulink-PS Converter/1
  connections:
  SADA/LConn2 -- +/RConn1
  Simulink-PS Converter/RConn1 -- SADA/LConn1
  SADA/RConn2 -- "- "/RConn1
  SADA/LConn3 -- -/RConn1
  SADA/RConn1 -- "+ "/RConn1

== system Two_Zone_MVDC_PSolver_R2020b/SCDD ==
  SADA : ee_lib/Switches & Breakers/DPST Switch  R_closed=1e-4 Ohm  G_open=1e-6 S  Threshold=0.5 V  Width=0 V  model_dynamics=0  t_on=1e-3 s  t_off=1e-3 s  initial_vT=0 V
      settings: SourceProductBaseCode=PS  InternalSimscapePortConfiguration="{\"Bottom\":[],\"Left\":[{\"id\":\"vT\",\"label\":\"vT\",\"type\":\"input\"},{\"id\":\"p1\",\"label\":\"\",\"type\":\"foundation.electrical.electrical\"},{\"id\":\"p2\",\"label\":\"\",\"type\":\"foundation.electrical.electrical\"}],\"Right\":[{\"id\":\"n1\",\"label\":\"\",\"type\":\"foundation.electrical.electrical\"},{\"id\":\"n2\",\"label\":\"\",\"type\":\"foundation.electrical.electrical\"}],\"Top\":[]}"
  Simulink-PS Converter : nesl_utility/Simulink-PS Converter  PhysicalDomain=network_engine_domain  SubClassName=ps_input  LeftPortType=input  RightPortType=output  PseudoPeriodic=off  Frequencies=[]  NoiseDistribution=none  NoiseParameters=[]  Unit=1  AffineConversion=off  FilteringAndDerivatives=provide  SimscapeFilterOrder=1  InputFilterTimeConstant=0.001  UdotUserProvided=0
  "+ " : PMIOPort  Side=Right
  + : PMIOPort  Port=2  Side=Left
  "- " : PMIOPort  Port=3  Side=Right
  - : PMIOPort  Port=4  Side=Left
  wires:
  [SCDD] -> Simulink-PS Converter/1
  connections:
  SADA/RConn1 -- "+ "/RConn1
  SADA/LConn3 -- -/RConn1
  SADA/RConn2 -- "- "/RConn1
  Simulink-PS Converter/RConn1 -- SADA/LConn1
  SADA/LConn2 -- +/RConn1

== system Two_Zone_MVDC_PSolver_R2020b/SDDA ==
  SDDA : ee_lib/Switches & Breakers/DPST Switch  R_closed=1e-4 Ohm  G_open=1e-6 S  Threshold=0.5 V  Width=0 V  model_dynamics=0  t_on=1e-3 s  t_off=1e-3 s  initial_vT=0 V
      settings: SourceProductBaseCode=PS  InternalSimscapePortConfiguration="{\"Bottom\":[],\"Left\":[{\"id\":\"vT\",\"label\":\"vT\",\"type\":\"input\"},{\"id\":\"p1\",\"label\":\"\",\"type\":\"foundation.electrical.electrical\"},{\"id\":\"p2\",\"label\":\"\",\"type\":\"foundation.electrical.electrical\"}],\"Right\":[{\"id\":\"n1\",\"label\":\"\",\"type\":\"foundation.electrical.electrical\"},{\"id\":\"n2\",\"label\":\"\",\"type\":\"foundation.electrical.electrical\"}],\"Top\":[]}"
  Simulink-PS Converter : nesl_utility/Simulink-PS Converter  PhysicalDomain=network_engine_domain  SubClassName=ps_input  LeftPortType=input  RightPortType=output  PseudoPeriodic=off  Frequencies=[]  NoiseDistribution=none  NoiseParameters=[]  Unit=1  AffineConversion=off  FilteringAndDerivatives=provide  SimscapeFilterOrder=1  InputFilterTimeConstant=0.001  UdotUserProvided=0
  "+ " : PMIOPort  Side=Right
  + : PMIOPort  Port=2  Side=Left
  "- " : PMIOPort  Port=3  Side=Right
  - : PMIOPort  Port=4  Side=Left
  wires:
  [SDDA] -> Simulink-PS Converter/1
  connections:
  SDDA/LConn2 -- +/RConn1
  Simulink-PS Converter/RConn1 -- SDDA/LConn1
  SDDA/RConn2 -- "- "/RConn1
  SDDA/LConn3 -- -/RConn1
  SDDA/RConn1 -- "+ "/RConn1

== system Two_Zone_MVDC_PSolver_R2020b/SDDB ==
  SDDB : ee_lib/Switches & Breakers/DPST Switch  R_closed=1e-4 Ohm  G_open=1e-6 S  Threshold=0.5 V  Width=0 V  model_dynamics=0  t_on=1e-3 s  t_off=1e-3 s  initial_vT=0 V
      settings: SourceProductBaseCode=PS  InternalSimscapePortConfiguration="{\"Bottom\":[],\"Left\":[{\"id\":\"vT\",\"label\":\"vT\",\"type\":\"input\"},{\"id\":\"p1\",\"label\":\"\",\"type\":\"foundation.electrical.electrical\"},{\"id\":\"p2\",\"label\":\"\",\"type\":\"foundation.electrical.electrical\"}],\"Right\":[{\"id\":\"n1\",\"label\":\"\",\"type\":\"foundation.electrical.electrical\"},{\"id\":\"n2\",\"label\":\"\",\"type\":\"foundation.electrical.electrical\"}],\"Top\":[]}"
  Simulink-PS Converter : nesl_utility/Simulink-PS Converter  PhysicalDomain=network_engine_domain  SubClassName=ps_input  LeftPortType=input  RightPortType=output  PseudoPeriodic=off  Frequencies=[]  NoiseDistribution=none  NoiseParameters=[]  Unit=1  AffineConversion=off  FilteringAndDerivatives=provide  SimscapeFilterOrder=1  InputFilterTimeConstant=0.001  UdotUserProvided=0
  "+ " : PMIOPort  Side=Right
  + : PMIOPort  Port=2  Side=Left
  "- " : PMIOPort  Port=3  Side=Right
  - : PMIOPort  Port=4  Side=Left
  wires:
  [SDDB] -> Simulink-PS Converter/1
  connections:
  SDDB/RConn1 -- "+ "/RConn1
  SDDB/LConn3 -- -/RConn1
  SDDB/RConn2 -- "- "/RConn1
  Simulink-PS Converter/RConn1 -- SDDB/LConn1
  SDDB/LConn2 -- +/RConn1

== system Two_Zone_MVDC_PSolver_R2020b/SDDC ==
  SDDC : ee_lib/Switches & Breakers/DPST Switch  R_closed=1e-4 Ohm  G_open=1e-6 S  Threshold=0.5 V  Width=0 V  model_dynamics=0  t_on=1e-3 s  t_off=1e-3 s  initial_vT=0 V
      settings: SourceProductBaseCode=PS  InternalSimscapePortConfiguration="{\"Bottom\":[],\"Left\":[{\"id\":\"vT\",\"label\":\"vT\",\"type\":\"input\"},{\"id\":\"p1\",\"label\":\"\",\"type\":\"foundation.electrical.electrical\"},{\"id\":\"p2\",\"label\":\"\",\"type\":\"foundation.electrical.electrical\"}],\"Right\":[{\"id\":\"n1\",\"label\":\"\",\"type\":\"foundation.electrical.electrical\"},{\"id\":\"n2\",\"label\":\"\",\"type\":\"foundation.electrical.electrical\"}],\"Top\":[]}"
  Simulink-PS Converter : nesl_utility/Simulink-PS Converter  PhysicalDomain=network_engine_domain  SubClassName=ps_input  LeftPortType=input  RightPortType=output  PseudoPeriodic=off  Frequencies=[]  NoiseDistribution=none  NoiseParameters=[]  Unit=1  AffineConversion=off  FilteringAndDerivatives=provide  SimscapeFilterOrder=1  InputFilterTimeConstant=0.001  UdotUserProvided=0
  "+ " : PMIOPort  Side=Right
  + : PMIOPort  Port=2  Side=Left
  "- " : PMIOPort  Port=3  Side=Right
  - : PMIOPort  Port=4  Side=Left
  wires:
  [SDDC] -> Simulink-PS Converter/1
  connections:
  SDDC/LConn2 -- +/RConn1
  Simulink-PS Converter/RConn1 -- SDDC/LConn1
  SDDC/RConn2 -- "- "/RConn1
  SDDC/LConn3 -- -/RConn1
  SDDC/RConn1 -- "+ "/RConn1

== system Two_Zone_MVDC_PSolver_R2020b/SDDD ==
  SDDD : ee_lib/Switches & Breakers/DPST Switch  R_closed=1e-4 Ohm  G_open=1e-6 S  Threshold=0.5 V  Width=0 V  model_dynamics=0  t_on=1e-3 s  t_off=1e-3 s  initial_vT=0 V
      settings: SourceProductBaseCode=PS  InternalSimscapePortConfiguration="{\"Bottom\":[],\"Left\":[{\"id\":\"vT\",\"label\":\"vT\",\"type\":\"input\"},{\"id\":\"p1\",\"label\":\"\",\"type\":\"foundation.electrical.electrical\"},{\"id\":\"p2\",\"label\":\"\",\"type\":\"foundation.electrical.electrical\"}],\"Right\":[{\"id\":\"n1\",\"label\":\"\",\"type\":\"foundation.electrical.electrical\"},{\"id\":\"n2\",\"label\":\"\",\"type\":\"foundation.electrical.electrical\"}],\"Top\":[]}"
  Simulink-PS Converter : nesl_utility/Simulink-PS Converter  PhysicalDomain=network_engine_domain  SubClassName=ps_input  LeftPortType=input  RightPortType=output  PseudoPeriodic=off  Frequencies=[]  NoiseDistribution=none  NoiseParameters=[]  Unit=1  AffineConversion=off  FilteringAndDerivatives=provide  SimscapeFilterOrder=1  InputFilterTimeConstant=0.001  UdotUserProvided=0
  "+ " : PMIOPort  Side=Right
  + : PMIOPort  Port=2  Side=Left
  "- " : PMIOPort  Port=3  Side=Right
  - : PMIOPort  Port=4  Side=Left
  wires:
  [SDDD] -> Simulink-PS Converter/1
  connections:
  SDDD/RConn1 -- "+ "/RConn1
  SDDD/LConn3 -- -/RConn1
  SDDD/RConn2 -- "- "/RConn1
  Simulink-PS Converter/RConn1 -- SDDD/LConn1
  SDDD/LConn2 -- +/RConn1

== system Two_Zone_MVDC_PSolver_R2020b/SDDE ==
  SDDE : ee_lib/Switches & Breakers/DPST Switch  R_closed=1e-4 Ohm  G_open=1e-6 S  Threshold=0.5 V  Width=0 V  model_dynamics=0  t_on=1e-3 s  t_off=1e-3 s  initial_vT=0 V
      settings: SourceProductBaseCode=PS  InternalSimscapePortConfiguration="{\"Bottom\":[],\"Left\":[{\"id\":\"vT\",\"label\":\"vT\",\"type\":\"input\"},{\"id\":\"p1\",\"label\":\"\",\"type\":\"foundation.electrical.electrical\"},{\"id\":\"p2\",\"label\":\"\",\"type\":\"foundation.electrical.electrical\"}],\"Right\":[{\"id\":\"n1\",\"label\":\"\",\"type\":\"foundation.electrical.electrical\"},{\"id\":\"n2\",\"label\":\"\",\"type\":\"foundation.electrical.electrical\"}],\"Top\":[]}"
  Simulink-PS Converter : nesl_utility/Simulink-PS Converter  PhysicalDomain=network_engine_domain  SubClassName=ps_input  LeftPortType=input  RightPortType=output  PseudoPeriodic=off  Frequencies=[]  NoiseDistribution=none  NoiseParameters=[]  Unit=1  AffineConversion=off  FilteringAndDerivatives=provide  SimscapeFilterOrder=1  InputFilterTimeConstant=0.001  UdotUserProvided=0
  "+ " : PMIOPort  Side=Right
  + : PMIOPort  Port=2  Side=Left
  "- " : PMIOPort  Port=3  Side=Right
  - : PMIOPort  Port=4  Side=Left
  wires:
  [SDDE] -> Simulink-PS Converter/1
  connections:
  SDDE/RConn1 -- "+ "/RConn1
  SDDE/LConn3 -- -/RConn1
  SDDE/RConn2 -- "- "/RConn1
  Simulink-PS Converter/RConn1 -- SDDE/LConn1
  SDDE/LConn2 -- +/RConn1

== system Two_Zone_MVDC_PSolver_R2020b/Subsystem1 ==
  Inductor1 : fl_lib/Electrical/Electrical Elements/Inductor  l=5.32e-6 H  r=0.32e-3 Ohm  g=0 1/Ohm  i_specify=off  i_priority=None  i=0 A  i_nominal_specify=off  i_nominal_unit=A  i_nominal_value=1  v_specify=off  v_priority=None  v=0 V  v_nominal_specify=off  v_nominal_unit=V  v_nominal_value=1  i_L_specify=off  i_L_priority=High  i_L=0 A  i_L_nominal_specify=off  i_L_nominal_unit=A  i_L_nominal_value=1
  Inductor2 : fl_lib/Electrical/Electrical Elements/Inductor  l=5.32e-6 H  r=0.32e-3 Ohm  g=0 1/Ohm  i_specify=off  i_priority=None  i=0 A  i_nominal_specify=off  i_nominal_unit=A  i_nominal_value=1  v_specify=off  v_priority=None  v=0 V  v_nominal_specify=off  v_nominal_unit=V  v_nominal_value=1  i_L_specify=off  i_L_priority=High  i_L=0 A  i_L_nominal_specify=off  i_L_nominal_unit=A  i_L_nominal_value=1
  Resistor : fl_lib/Electrical/Electrical Elements/Resistor  R=Rsnub Ohm  i_specify=off  i_priority=None  i=0 A  i_nominal_specify=off  i_nominal_unit=A  i_nominal_value=1  v_specify=off  v_priority=None  v=0 V  v_nominal_specify=off  v_nominal_unit=V  v_nominal_value=1
  Resistor1 : fl_lib/Electrical/Electrical Elements/Resistor  R=Rsnub Ohm  i_specify=off  i_priority=None  i=0 A  i_nominal_specify=off  i_nominal_unit=A  i_nominal_value=1  v_specify=off  v_priority=None  v=0 V  v_nominal_specify=off  v_nominal_unit=V  v_nominal_value=1
  "+ " : PMIOPort  Side=Left
  + : PMIOPort  Port=2  Side=Right
  - : PMIOPort  Port=3  Side=Left
  "- " : PMIOPort  Port=4  Side=Right
  connections:
  Inductor1/LConn1 -- Resistor/RConn1 -- -/RConn1
  Inductor2/LConn1 -- Resistor/LConn1 -- "+ "/RConn1
  Inductor2/RConn1 -- Resistor1/LConn1 -- +/RConn1
  Inductor1/RConn1 -- Resistor1/RConn1 -- "- "/RConn1

== system Two_Zone_MVDC_PSolver_R2020b/Subsystem10 ==
  Current Sensor : fl_lib/Electrical/Electrical Sensors/Current Sensor
  Inductor1 : fl_lib/Electrical/Electrical Elements/Inductor  l=3.47e-6 H  r=0.21e-3 Ohm  g=0 1/Ohm  i_specify=off  i_priority=None  i=0 A  i_nominal_specify=off  i_nominal_unit=A  i_nominal_value=1  v_specify=off  v_priority=None  v=0 V  v_nominal_specify=off  v_nominal_unit=V  v_nominal_value=1  i_L_specify=off  i_L_priority=High  i_L=0 A  i_L_nominal_specify=off  i_L_nominal_unit=A  i_L_nominal_value=1
  Inductor3 : fl_lib/Electrical/Electrical Elements/Inductor  l=3.47e-6 H  r=0.21e-3 Ohm  g=0 1/Ohm  i_specify=off  i_priority=None  i=0 A  i_nominal_specify=off  i_nominal_unit=A  i_nominal_value=1  v_specify=off  v_priority=None  v=0 V  v_nominal_specify=off  v_nominal_unit=V  v_nominal_value=1  i_L_specify=off  i_L_priority=High  i_L=0 A  i_L_nominal_specify=off  i_L_nominal_unit=A  i_L_nominal_value=1
  PS-Simulink Converter : nesl_utility/PS-Simulink Converter  PhysicalDomain=network_engine_domain  SubClassName=ps_output  LeftPortType=input  RightPortType=output  PseudoPeriodic=off  Frequencies=[]  Unit=inherit  AffineConversion=off
  PS-Simulink Converter1 : nesl_utility/PS-Simulink Converter  PhysicalDomain=network_engine_domain  SubClassName=ps_output  LeftPortType=input  RightPortType=output  PseudoPeriodic=off  Frequencies=[]  Unit=inherit  AffineConversion=off
  Product : Product
  Resistor : fl_lib/Electrical/Electrical Elements/Resistor  R=Rsnub Ohm  i_specify=off  i_priority=None  i=0 A  i_nominal_specify=off  i_nominal_unit=A  i_nominal_value=1  v_specify=off  v_priority=None  v=0 V  v_nominal_specify=off  v_nominal_unit=V  v_nominal_value=1
  Terminator : Terminator
  Voltage Sensor : fl_lib/Electrical/Electrical Sensors/Voltage Sensor
  "+ " : PMIOPort  Side=Left
  + : PMIOPort  Port=2  Side=Right
  - : PMIOPort  Port=3  Side=Left
  "- " : PMIOPort  Port=4  Side=Right
  wires:
  Product/1 -> Terminator/1  "P_CS6"
  PS-Simulink Converter/1 -> Product/1
  PS-Simulink Converter1/1 -> Product/2
  connections:
  Inductor1/LConn1 -- Resistor/RConn1 -- -/RConn1
  Inductor3/LConn1 -- Resistor/LConn1 -- "+ "/RConn1
  Inductor3/RConn1 -- Current Sensor/LConn1
  Current Sensor/RConn2 -- Voltage Sensor/LConn1 -- +/RConn1
  Inductor1/RConn1 -- Voltage Sensor/RConn2 -- "- "/RConn1
  Voltage Sensor/RConn1 -- PS-Simulink Converter1/LConn1
  PS-Simulink Converter/LConn1 -- Current Sensor/RConn1
